simulink model "parrotMinidroneWaypointFollower"  (R2020a)
settings: Solver=ode3  StartTime=0  StopTime=TFinal  FixedStep=Ts  RelTol=1e-3  EnableMultiTasking=on
undefined symbols (not defined in the file): Command, Fault_Category, ft, gcbh, init, m, Rec, s, SDTV, sensorCalibrationData, Sensors, sigbuilder_block, States, stop_time, takeOffDuration, Ts, Vehicle, vrmfunc, VTs
libraries: simulink x16, aerolibconvert2 x4, environmentLibrary x2, visionconversions x2, visiongeotforms x2, aerolibutil x2, aerolibanimutils x1, aerolibnav x1, vrlib x1
(part 4 of 5)

== system parrotMinidroneWaypointFollower/Sensors Model/Sensors (Dynamics)/Sensor System/IMU_Pressure/HAL_acquisition_creator/Gyr Fault Injector1/GyrFI3 ==
  Gyr z : Inport
  Iflag : Inport  Port=2
  Cast To Double : DataTypeConversion  OutDataTypeStr=double
  Cast To Single : DataTypeConversion  OutDataTypeStr=single
  FIBlock : Subsystem  TreatAsAtomicUnit=on  mask(Fault Injector Block){FIBlockName=6, FInjEnable=off, FaultType=Bias/Offset, FaultValue=5, FaultEvent=Deterministic, EventValue=3, FaultEffect=Constant time, EffectValue=2}
      mask prompts: FIBlockName "Number of the FI block instance (e.i. 'name' of the fault injector)"; FInjEnable "Turn on the fault injection for this block"; FaultType "Fault type"; FaultValue "Fault value (bias)"; FaultEvent "Fault injection method"; EventValue "Event value (s)"; FaultEffect "Fault injection effect"; EffectValue "Effect value (s)"
      mask help:
      | This block allows to conduct a fault injection experiment (refer to help if needed).
      | Specify:
      | - name of the block instance.
      | - type of fault: Stuck-at, Package drop, Bias/Offset, Bit flips, Time delay, Noise.
      | - fault event: Failure probability, Mean Time to Failure, Failure Rate Distribution, Deterministic.
      | - fault effect: Once, Constant time, Infinite time, Mean Time to Repair.
      mask init: same as parrotMinidroneWaypointFollower/Sensors Model/Sensors (Dynamics)/Sensor System/IMU_Pressure/HAL_acquisition_creator/Acc Fault Injector/AccFI1/FIBlock
      mask Help:
      | Failure rate distribution is not supported yet!
      | Bit flips, Time delay, and Noise faults may have some bugs :D
      | In different FIBlock instances, the 'name' of the block in GUI must be different (must be an integer number).
      | 
      | Please refer to a comprehensive article regarding the FIBLock: https://flatag.tech/fiblock.html
      | Please cite as: "Fabarisov, T. et al. "Model-based Fault Injection Experiments for the Safety Analysis of Exoskeleton System." Proceedings of the 30th European Safety and Reliability Conference and the 15th Probabilistic Safety Assessment and Management Conference, 2020."
      | 
      | This block allows to conduct a fault injection experiment.
      | Specify:
      | 1) number of the block instance (e.i. 'name' of the fault injector, name shall be unique).
      | 
      | 2) type of fault:
      | - Stuck-at. The block output stays constant, preserving the latest correct value before the error occurrence.
      | - Package drop. The correct output is replaced by the specified Value, emulating a package drop.
      | - Bias/Offset . The defined positive or negative Bias value is added to the block output.
      | - Noise. A random noise value is added. The Boundaries are defined as the percentage of the correct value.
      | - Time delay. A delay is introduced into the signal. During the delay the value is zero.
      | - Bit flips. The defined Number of bits are inverted in the binary representation of the correct value.
      | 
      | 3) fault event:
      | - Failure probability. Errors are injected based on the constant Failure probability for each execution of the block function.
      | - Mean Time to Failure. Errors are injected according to the specified MTTF. Normal distribution.
      | - Deterministic. Уrrors are injected at specific time step.
      | 
      | 4) fault effect:
      | - Once. An error appears only one time during a simulation.
      | - Constant time. The block produces erroneous output during the specified Time period.
      | - Infinite time. The block produces erroneous output until the end of the simulation.
      | - Mean Time to Repair. Normally distributed MTTR regulates the time of the error effect.
      | 
      | FIBlock also provide, what we call, a chained fault injection.
      | Second output of the FIBlock emits a trigger flag.
      | This output signal could be connected to the second input of the FIBlock.
      | In case of the fault injection, this signal will force trigger fault injectionin second FIBlock.
      | 
      | FIBlock supports a base Workspace variables as input in the GUI parameters.
      | 
      | Made By Tagir Fabarisov, TU Dresden 2020
      mask TypeOptions FaultType: Stuck-at | Package drop | Bias/Offset | Bit flips | Time delay | Noise
      mask TypeOptions FaultEvent: Failure probability | Mean Time To Failure | Deterministic
      mask TypeOptions FaultEffect: Once | Constant time | Infinite time | Mean Time To Repair
      mask DialogControl FInjEnable Tooltip: If ticked, then this FIBlock will inject faults
      mask DialogControl Container8 Prompt: Fault type
      mask DialogControl FaultType Tooltip: Specify a type of fault that will be injected
      mask DialogControl FaultTypeDesc Prompt: The defined positive or negative Bias value is added to the block output.
      mask DialogControl Container3 Prompt: Fault injection method
      mask DialogControl Container6 Prompt: Event
      mask DialogControl FaultEvent Tooltip: Specify when fault will be injected
      mask DialogControl FaultEventDesc Prompt: Errors are injected at the specified time
      mask DialogControl Container7 Prompt: Effect
      mask DialogControl FaultEffect Tooltip: Specify how long fault will be injected
      mask DialogControl FaultEffectDesc Prompt: The block produces erroneous output during the specified Time period.
      mask Display:
      | warning off;
      | color('red');
      | a = FaultType;
      | if a == "Sensor: Stuck-at fault"
      |     color('black');
      |     x = linspace(-pi,pi);
      |     y = sin(x);
      |     plot(x,y);
      |     color('red');
      |     disp('        ↯');
      |     x = [-0.7 2];
      |     y = [-0.7 -0.7];
      |     plot(x,y);
      | elseif a == "Network: Package drop"
      |     color('black');
      |     x = linspace(-pi,pi);
      |     y = sin(x);
      |     plot(x,y);
      |     color('red');
      |     disp('        ↯');
      |     x = [-0.7 -0.7];
      |     y = [-0.7 0];
      |     plot(x,y);
      |     x = [-0.7 1];
      |     y = [0 0];
      |     plot(x,y);
      | elseif a == "Sensor: Offset"
      |     color('black');
      |     x1 = linspace(-pi,pi);
      |     y1 = sin(x1)-0.5;
      |     plot(x1,y1);
      |     color('red');
      |     disp('        ↯');
      |     x2 = linspace(0,pi);
      |     y2 = sin(x2);
      |     plot(x2,y2);
      |     x = [0 0];
      |     y = [-0.5 0];
      |     plot(x,y);
      | elseif a == "Hardware: Bit flips"
      |     color('black');
      |     disp('10101010');
      |     color('red');
      |     disp('    0↯');
      | elseif a == "Network: Time delay"
      |     color('black');
      |     x1 = linspace(-pi,pi);
      |     y1 = sin(x1);
      |     plot(x1,y1);
      |     color('red');
      |     disp('        ↯');
      |     x2 = linspace(0,pi);
      |     y2 = sin(x2-0.5);
      |     plot(x2,y2);
      |     x = [0 -0.4];
      |     y = [-0.5 -0.5];
      |     plot(x,y);
      | elseif a == "Sensor: Noise"
      |     color('black');
      |     x1 = linspace(-pi,pi);
      |     y1 = sin(x1);
      |     plot(x1,y1);
      |     color('red');
      |     disp('        ↯');
      |     x = linspace(-pi/8,pi/8,10);
      |     y = sin(x);
      |     for yc = 1:length(y)
      |         d = randi([-2,2])/5;
      |         y(yc) = y(yc) + d;
      |     end
      |     plot(x,y);
      | else
      |     color('red');
      |     disp('Set up Fault Injector!');
      | %Bit flips
      | %Time delay
      | %Noise
      | end
      | warning on;
  z : Outport
  Fflag : Outport  Port=2
  wires:
  Gyr z/1 -> Cast To Double/1
  FIBlock/1(Fdata) -> Cast To Single/1
  Cast To Double/1 -> FIBlock/1(Idata)
  Iflag/1 -> FIBlock/2(Iflag)
  Cast To Single/1 -> z/1
  FIBlock/2(Fflag) -> Fflag/1

== system parrotMinidroneWaypointFollower/Sensors Model/Sensors (Dynamics)/Sensor System/IMU_Pressure/HAL_acquisition_creator/Gyr Fault Injector2/GyrFI1 ==
  Gyr x : Inport
  Iflag : Inport  Port=2
  Cast To Double : DataTypeConversion  OutDataTypeStr=double
  Cast To Single : DataTypeConversion  OutDataTypeStr=single
  FIBlock : Subsystem  TreatAsAtomicUnit=on  mask(Fault Injector Block){FIBlockName=4, FInjEnable=on, FaultType=Bias/Offset, FaultValue=6, FaultEvent=Deterministic, EventValue=4, FaultEffect=Constant time, EffectValue=1.5}
      mask prompts: FIBlockName "Number of the FI block instance (e.i. 'name' of the fault injector)"; FInjEnable "Turn on the fault injection for this block"; FaultType "Fault type"; FaultValue "Fault value (bias)"; FaultEvent "Fault injection method"; EventValue "Event value (s)"; FaultEffect "Fault injection effect"; EffectValue "Effect value (s)"
      mask help:
      | This block allows to conduct a fault injection experiment (refer to help if needed).
      | Specify:
      | - name of the block instance.
      | - type of fault: Stuck-at, Package drop, Bias/Offset, Bit flips, Time delay, Noise.
      | - fault event: Failure probability, Mean Time to Failure, Failure Rate Distribution, Deterministic.
      | - fault effect: Once, Constant time, Infinite time, Mean Time to Repair.
      mask init: same as parrotMinidroneWaypointFollower/Sensors Model/Sensors (Dynamics)/Sensor System/IMU_Pressure/HAL_acquisition_creator/Acc Fault Injector/AccFI1/FIBlock
      mask Help:
      | Failure rate distribution is not supported yet!
      | Bit flips, Time delay, and Noise faults may have some bugs :D
      | In different FIBlock instances, the 'name' of the block in GUI must be different (must be an integer number).
      | 
      | Please refer to a comprehensive article regarding the FIBLock: https://flatag.tech/fiblock.html
      | Please cite as: "Fabarisov, T. et al. "Model-based Fault Injection Experiments for the Safety Analysis of Exoskeleton System." Proceedings of the 30th European Safety and Reliability Conference and the 15th Probabilistic Safety Assessment and Management Conference, 2020."
      | 
      | This block allows to conduct a fault injection experiment.
      | Specify:
      | 1) number of the block instance (e.i. 'name' of the fault injector, name shall be unique).
      | 
      | 2) type of fault:
      | - Stuck-at. The block output stays constant, preserving the latest correct value before the error occurrence.
      | - Package drop. The correct output is replaced by the specified Value, emulating a package drop.
      | - Bias/Offset . The defined positive or negative Bias value is added to the block output.
      | - Noise. A random noise value is added. The Boundaries are defined as the percentage of the correct value.
      | - Time delay. A delay is introduced into the signal. During the delay the value is zero.
      | - Bit flips. The defined Number of bits are inverted in the binary representation of the correct value.
      | 
      | 3) fault event:
      | - Failure probability. Errors are injected based on the constant Failure probability for each execution of the block function.
      | - Mean Time to Failure. Errors are injected according to the specified MTTF. Normal distribution.
      | - Deterministic. Уrrors are injected at specific time step.
      | 
      | 4) fault effect:
      | - Once. An error appears only one time during a simulation.
      | - Constant time. The block produces erroneous output during the specified Time period.
      | - Infinite time. The block produces erroneous output until the end of the simulation.
      | - Mean Time to Repair. Normally distributed MTTR regulates the time of the error effect.
      | 
      | FIBlock also provide, what we call, a chained fault injection.
      | Second output of the FIBlock emits a trigger flag.
      | This output signal could be connected to the second input of the FIBlock.
      | In case of the fault injection, this signal will force trigger fault injectionin second FIBlock.
      | 
      | FIBlock supports a base Workspace variables as input in the GUI parameters.
      | 
      | Made By Tagir Fabarisov, TU Dresden 2020
      mask TypeOptions FaultType: Stuck-at | Package drop | Bias/Offset | Bit flips | Time delay | Noise
      mask TypeOptions FaultEvent: Failure probability | Mean Time To Failure | Deterministic
      mask TypeOptions FaultEffect: Once | Constant time | Infinite time | Mean Time To Repair
      mask DialogControl FInjEnable Tooltip: If ticked, then this FIBlock will inject faults
      mask DialogControl Container8 Prompt: Fault type
      mask DialogControl FaultType Tooltip: Specify a type of fault that will be injected
      mask DialogControl FaultTypeDesc Prompt: The defined positive or negative Bias value is added to the block output.
      mask DialogControl Container3 Prompt: Fault injection method
      mask DialogControl Container6 Prompt: Event
      mask DialogControl FaultEvent Tooltip: Specify when fault will be injected
      mask DialogControl FaultEventDesc Prompt: Errors are injected at the specified time
      mask DialogControl Container7 Prompt: Effect
      mask DialogControl FaultEffect Tooltip: Specify how long fault will be injected
      mask DialogControl FaultEffectDesc Prompt: The block produces erroneous output during the specified Time period.
      mask Display:
      | warning off;
      | color('red');
      | a = FaultType;
      | if a == "Sensor: Stuck-at fault"
      |     color('black');
      |     x = linspace(-pi,pi);
      |     y = sin(x);
      |     plot(x,y);
      |     color('red');
      |     disp('        ↯');
      |     x = [-0.7 2];
      |     y = [-0.7 -0.7];
      |     plot(x,y);
      | elseif a == "Network: Package drop"
      |     color('black');
      |     x = linspace(-pi,pi);
      |     y = sin(x);
      |     plot(x,y);
      |     color('red');
      |     disp('        ↯');
      |     x = [-0.7 -0.7];
      |     y = [-0.7 0];
      |     plot(x,y);
      |     x = [-0.7 1];
      |     y = [0 0];
      |     plot(x,y);
      | elseif a == "Sensor: Offset"
      |     color('black');
      |     x1 = linspace(-pi,pi);
      |     y1 = sin(x1)-0.5;
      |     plot(x1,y1);
      |     color('red');
      |     disp('        ↯');
      |     x2 = linspace(0,pi);
      |     y2 = sin(x2);
      |     plot(x2,y2);
      |     x = [0 0];
      |     y = [-0.5 0];
      |     plot(x,y);
      | elseif a == "Hardware: Bit flips"
      |     color('black');
      |     disp('10101010');
      |     color('red');
      |     disp('    0↯');
      | elseif a == "Network: Time delay"
      |     color('black');
      |     x1 = linspace(-pi,pi);
      |     y1 = sin(x1);
      |     plot(x1,y1);
      |     color('red');
      |     disp('        ↯');
      |     x2 = linspace(0,pi);
      |     y2 = sin(x2-0.5);
      |     plot(x2,y2);
      |     x = [0 -0.4];
      |     y = [-0.5 -0.5];
      |     plot(x,y);
      | elseif a == "Sensor: Noise"
      |     color('black');
      |     x1 = linspace(-pi,pi);
      |     y1 = sin(x1);
      |     plot(x1,y1);
      |     color('red');
      |     disp('        ↯');
      |     x = linspace(-pi/8,pi/8,10);
      |     y = sin(x);
      |     for yc = 1:length(y)
      |         d = randi([-2,2])/5;
      |         y(yc) = y(yc) + d;
      |     end
      |     plot(x,y);
      | else
      |     color('red');
      |     disp('Set up Fault Injector!');
      | %Bit flips
      | %Time delay
      | %Noise
      | end
      | warning on;
  Fflag : Outport
  x : Outport  Port=2
  wires:
  Gyr x/1 -> Cast To Double/1
  FIBlock/1(Fdata) -> Cast To Single/1
  Cast To Double/1 -> FIBlock/1(Idata)
  Iflag/1 -> FIBlock/2(Iflag)
  Cast To Single/1 -> x/1
  FIBlock/2(Fflag) -> Fflag/1

== system parrotMinidroneWaypointFollower/Sensors Model/Sensors (Dynamics)/Sensor System/IMU_Pressure/HAL_acquisition_creator/Gyr Fault Injector2/GyrFI2 ==
  Gyr y : Inport
  Iflag : Inport  Port=2
  Cast To Double : DataTypeConversion  OutDataTypeStr=double
  Cast To Single : DataTypeConversion  OutDataTypeStr=single
  FIBlock : Subsystem  TreatAsAtomicUnit=on  mask(Fault Injector Block){FIBlockName=5, FInjEnable=off, FaultType=Bias/Offset, FaultValue=6, FaultEvent=Deterministic, EventValue=3, FaultEffect=Constant time, EffectValue=2}
      mask prompts: FIBlockName "Number of the FI block instance (e.i. 'name' of the fault injector)"; FInjEnable "Turn on the fault injection for this block"; FaultType "Fault type"; FaultValue "Fault value (bias)"; FaultEvent "Fault injection method"; EventValue "Event value (s)"; FaultEffect "Fault injection effect"; EffectValue "Effect value (s)"
      mask help:
      | This block allows to conduct a fault injection experiment (refer to help if needed).
      | Specify:
      | - name of the block instance.
      | - type of fault: Stuck-at, Package drop, Bias/Offset, Bit flips, Time delay, Noise.
      | - fault event: Failure probability, Mean Time to Failure, Failure Rate Distribution, Deterministic.
      | - fault effect: Once, Constant time, Infinite time, Mean Time to Repair.
      mask init: same as parrotMinidroneWaypointFollower/Sensors Model/Sensors (Dynamics)/Sensor System/IMU_Pressure/HAL_acquisition_creator/Acc Fault Injector/AccFI1/FIBlock
      mask Help:
      | Failure rate distribution is not supported yet!
      | Bit flips, Time delay, and Noise faults may have some bugs :D
      | In different FIBlock instances, the 'name' of the block in GUI must be different (must be an integer number).
      | 
      | Please refer to a comprehensive article regarding the FIBLock: https://flatag.tech/fiblock.html
      | Please cite as: "Fabarisov, T. et al. "Model-based Fault Injection Experiments for the Safety Analysis of Exoskeleton System." Proceedings of the 30th European Safety and Reliability Conference and the 15th Probabilistic Safety Assessment and Management Conference, 2020."
      | 
      | This block allows to conduct a fault injection experiment.
      | Specify:
      | 1) number of the block instance (e.i. 'name' of the fault injector, name shall be unique).
      | 
      | 2) type of fault:
      | - Stuck-at. The block output stays constant, preserving the latest correct value before the error occurrence.
      | - Package drop. The correct output is replaced by the specified Value, emulating a package drop.
      | - Bias/Offset . The defined positive or negative Bias value is added to the block output.
      | - Noise. A random noise value is added. The Boundaries are defined as the percentage of the correct value.
      | - Time delay. A delay is introduced into the signal. During the delay the value is zero.
      | - Bit flips. The defined Number of bits are inverted in the binary representation of the correct value.
      | 
      | 3) fault event:
      | - Failure probability. Errors are injected based on the constant Failure probability for each execution of the block function.
      | - Mean Time to Failure. Errors are injected according to the specified MTTF. Normal distribution.
      | - Deterministic. Уrrors are injected at specific time step.
      | 
      | 4) fault effect:
      | - Once. An error appears only one time during a simulation.
      | - Constant time. The block produces erroneous output during the specified Time period.
      | - Infinite time. The block produces erroneous output until the end of the simulation.
      | - Mean Time to Repair. Normally distributed MTTR regulates the time of the error effect.
      | 
      | FIBlock also provide, what we call, a chained fault injection.
      | Second output of the FIBlock emits a trigger flag.
      | This output signal could be connected to the second input of the FIBlock.
      | In case of the fault injection, this signal will force trigger fault injectionin second FIBlock.
      | 
      | FIBlock supports a base Workspace variables as input in the GUI parameters.
      | 
      | Made By Tagir Fabarisov, TU Dresden 2020
      mask TypeOptions FaultType: Stuck-at | Package drop | Bias/Offset | Bit flips | Time delay | Noise
      mask TypeOptions FaultEvent: Failure probability | Mean Time To Failure | Deterministic
      mask TypeOptions FaultEffect: Once | Constant time | Infinite time | Mean Time To Repair
      mask DialogControl FInjEnable Tooltip: If ticked, then this FIBlock will inject faults
      mask DialogControl Container8 Prompt: Fault type
      mask DialogControl FaultType Tooltip: Specify a type of fault that will be injected
      mask DialogControl FaultTypeDesc Prompt: The defined positive or negative Bias value is added to the block output.
      mask DialogControl Container3 Prompt: Fault injection method
      mask DialogControl Container6 Prompt: Event
      mask DialogControl FaultEvent Tooltip: Specify when fault will be injected
      mask DialogControl FaultEventDesc Prompt: Errors are injected at the specified time
      mask DialogControl Container7 Prompt: Effect
      mask DialogControl FaultEffect Tooltip: Specify how long fault will be injected
      mask DialogControl FaultEffectDesc Prompt: The block produces erroneous output during the specified Time period.
      mask Display:
      | warning off;
      | color('red');
      | a = FaultType;
      | if a == "Sensor: Stuck-at fault"
      |     color('black');
      |     x = linspace(-pi,pi);
      |     y = sin(x);
      |     plot(x,y);
      |     color('red');
      |     disp('        ↯');
      |     x = [-0.7 2];
      |     y = [-0.7 -0.7];
      |     plot(x,y);
      | elseif a == "Network: Package drop"
      |     color('black');
      |     x = linspace(-pi,pi);
      |     y = sin(x);
      |     plot(x,y);
      |     color('red');
      |     disp('        ↯');
      |     x = [-0.7 -0.7];
      |     y = [-0.7 0];
      |     plot(x,y);
      |     x = [-0.7 1];
      |     y = [0 0];
      |     plot(x,y);
      | elseif a == "Sensor: Offset"
      |     color('black');
      |     x1 = linspace(-pi,pi);
      |     y1 = sin(x1)-0.5;
      |     plot(x1,y1);
      |     color('red');
      |     disp('        ↯');
      |     x2 = linspace(0,pi);
      |     y2 = sin(x2);
      |     plot(x2,y2);
      |     x = [0 0];
      |     y = [-0.5 0];
      |     plot(x,y);
      | elseif a == "Hardware: Bit flips"
      |     color('black');
      |     disp('10101010');
      |     color('red');
      |     disp('    0↯');
      | elseif a == "Network: Time delay"
      |     color('black');
      |     x1 = linspace(-pi,pi);
      |     y1 = sin(x1);
      |     plot(x1,y1);
      |     color('red');
      |     disp('        ↯');
      |     x2 = linspace(0,pi);
      |     y2 = sin(x2-0.5);
      |     plot(x2,y2);
      |     x = [0 -0.4];
      |     y = [-0.5 -0.5];
      |     plot(x,y);
      | elseif a == "Sensor: Noise"
      |     color('black');
      |     x1 = linspace(-pi,pi);
      |     y1 = sin(x1);
      |     plot(x1,y1);
      |     color('red');
      |     disp('        ↯');
      |     x = linspace(-pi/8,pi/8,10);
      |     y = sin(x);
      |     for yc = 1:length(y)
      |         d = randi([-2,2])/5;
      |         y(yc) = y(yc) + d;
      |     end
      |     plot(x,y);
      | else
      |     color('red');
      |     disp('Set up Fault Injector!');
      | %Bit flips
      | %Time delay
      | %Noise
      | end
      | warning on;
  Fflag : Outport
  y : Outport  Port=2
  wires:
  Gyr y/1 -> Cast To Double/1
  FIBlock/1(Fdata) -> Cast To Single/1
  Cast To Double/1 -> FIBlock/1(Idata)
  Iflag/1 -> FIBlock/2(Iflag)
  Cast To Single/1 -> y/1
  FIBlock/2(Fflag) -> Fflag/1

== system parrotMinidroneWaypointFollower/Sensors Model/Sensors (Dynamics)/Sensor System/IMU_Pressure/HAL_acquisition_creator/Gyr Fault Injector2/GyrFI3 ==
  Gyr z : Inport
  Iflag : Inport  Port=2
  Cast To Double : DataTypeConversion  OutDataTypeStr=double
  Cast To Single : DataTypeConversion  OutDataTypeStr=single
  FIBlock : Subsystem  TreatAsAtomicUnit=on  mask(Fault Injector Block){FIBlockName=6, FInjEnable=off, FaultType=Bias/Offset, FaultValue=5, FaultEvent=Deterministic, EventValue=3, FaultEffect=Constant time, EffectValue=2}
      mask prompts: FIBlockName "Number of the FI block instance (e.i. 'name' of the fault injector)"; FInjEnable "Turn on the fault injection for this block"; FaultType "Fault type"; FaultValue "Fault value (bias)"; FaultEvent "Fault injection method"; EventValue "Event value (s)"; FaultEffect "Fault injection effect"; EffectValue "Effect value (s)"
      mask help:
      | This block allows to conduct a fault injection experiment (refer to help if needed).
      | Specify:
      | - name of the block instance.
      | - type of fault: Stuck-at, Package drop, Bias/Offset, Bit flips, Time delay, Noise.
      | - fault event: Failure probability, Mean Time to Failure, Failure Rate Distribution, Deterministic.
      | - fault effect: Once, Constant time, Infinite time, Mean Time to Repair.
      mask init: same as parrotMinidroneWaypointFollower/Sensors Model/Sensors (Dynamics)/Sensor System/IMU_Pressure/HAL_acquisition_creator/Acc Fault Injector/AccFI1/FIBlock
      mask Help:
      | Failure rate distribution is not supported yet!
      | Bit flips, Time delay, and Noise faults may have some bugs :D
      | In different FIBlock instances, the 'name' of the block in GUI must be different (must be an integer number).
      | 
      | Please refer to a comprehensive article regarding the FIBLock: https://flatag.tech/fiblock.html
      | Please cite as: "Fabarisov, T. et al. "Model-based Fault Injection Experiments for the Safety Analysis of Exoskeleton System." Proceedings of the 30th European Safety and Reliability Conference and the 15th Probabilistic Safety Assessment and Management Conference, 2020."
      | 
      | This block allows to conduct a fault injection experiment.
      | Specify:
      | 1) number of the block instance (e.i. 'name' of the fault injector, name shall be unique).
      | 
      | 2) type of fault:
      | - Stuck-at. The block output stays constant, preserving the latest correct value before the error occurrence.
      | - Package drop. The correct output is replaced by the specified Value, emulating a package drop.
      | - Bias/Offset . The defined positive or negative Bias value is added to the block output.
      | - Noise. A random noise value is added. The Boundaries are defined as the percentage of the correct value.
      | - Time delay. A delay is introduced into the signal. During the delay the value is zero.
      | - Bit flips. The defined Number of bits are inverted in the binary representation of the correct value.
      | 
      | 3) fault event:
      | - Failure probability. Errors are injected based on the constant Failure probability for each execution of the block function.
      | - Mean Time to Failure. Errors are injected according to the specified MTTF. Normal distribution.
      | - Deterministic. Уrrors are injected at specific time step.
      | 
      | 4) fault effect:
      | - Once. An error appears only one time during a simulation.
      | - Constant time. The block produces erroneous output during the specified Time period.
      | - Infinite time. The block produces erroneous output until the end of the simulation.
      | - Mean Time to Repair. Normally distributed MTTR regulates the time of the error effect.
      | 
      | FIBlock also provide, what we call, a chained fault injection.
      | Second output of the FIBlock emits a trigger flag.
      | This output signal could be connected to the second input of the FIBlock.
      | In case of the fault injection, this signal will force trigger fault injectionin second FIBlock.
      | 
      | FIBlock supports a base Workspace variables as input in the GUI parameters.
      | 
      | Made By Tagir Fabarisov, TU Dresden 2020
      mask TypeOptions FaultType: Stuck-at | Package drop | Bias/Offset | Bit flips | Time delay | Noise
      mask TypeOptions FaultEvent: Failure probability | Mean Time To Failure | Deterministic
      mask TypeOptions FaultEffect: Once | Constant time | Infinite time | Mean Time To Repair
      mask DialogControl FInjEnable Tooltip: If ticked, then this FIBlock will inject faults
      mask DialogControl Container8 Prompt: Fault type
      mask DialogControl FaultType Tooltip: Specify a type of fault that will be injected
      mask DialogControl FaultTypeDesc Prompt: The defined positive or negative Bias value is added to the block output.
      mask DialogControl Container3 Prompt: Fault injection method
      mask DialogControl Container6 Prompt: Event
      mask DialogControl FaultEvent Tooltip: Specify when fault will be injected
      mask DialogControl FaultEventDesc Prompt: Errors are injected at the specified time
      mask DialogControl Container7 Prompt: Effect
      mask DialogControl FaultEffect Tooltip: Specify how long fault will be injected
      mask DialogControl FaultEffectDesc Prompt: The block produces erroneous output during the specified Time period.
      mask Display:
      | warning off;
      | color('red');
      | a = FaultType;
      | if a == "Sensor: Stuck-at fault"
      |     color('black');
      |     x = linspace(-pi,pi);
      |     y = sin(x);
      |     plot(x,y);
      |     color('red');
      |     disp('        ↯');
      |     x = [-0.7 2];
      |     y = [-0.7 -0.7];
      |     plot(x,y);
      | elseif a == "Network: Package drop"
      |     color('black');
      |     x = linspace(-pi,pi);
      |     y = sin(x);
      |     plot(x,y);
      |     color('red');
      |     disp('        ↯');
      |     x = [-0.7 -0.7];
      |     y = [-0.7 0];
      |     plot(x,y);
      |     x = [-0.7 1];
      |     y = [0 0];
      |     plot(x,y);
      | elseif a == "Sensor: Offset"
      |     color('black');
      |     x1 = linspace(-pi,pi);
      |     y1 = sin(x1)-0.5;
      |     plot(x1,y1);
      |     color('red');
      |     disp('        ↯');
      |     x2 = linspace(0,pi);
      |     y2 = sin(x2);
      |     plot(x2,y2);
      |     x = [0 0];
      |     y = [-0.5 0];
      |     plot(x,y);
      | elseif a == "Hardware: Bit flips"
      |     color('black');
      |     disp('10101010');
      |     color('red');
      |     disp('    0↯');
      | elseif a == "Network: Time delay"
      |     color('black');
      |     x1 = linspace(-pi,pi);
      |     y1 = sin(x1);
      |     plot(x1,y1);
      |     color('red');
      |     disp('        ↯');
      |     x2 = linspace(0,pi);
      |     y2 = sin(x2-0.5);
      |     plot(x2,y2);
      |     x = [0 -0.4];
      |     y = [-0.5 -0.5];
      |     plot(x,y);
      | elseif a == "Sensor: Noise"
      |     color('black');
      |     x1 = linspace(-pi,pi);
      |     y1 = sin(x1);
      |     plot(x1,y1);
      |     color('red');
      |     disp('        ↯');
      |     x = linspace(-pi/8,pi/8,10);
      |     y = sin(x);
      |     for yc = 1:length(y)
      |         d = randi([-2,2])/5;
      |         y(yc) = y(yc) + d;
      |     end
      |     plot(x,y);
      | else
      |     color('red');
      |     disp('Set up Fault Injector!');
      | %Bit flips
      | %Time delay
      | %Noise
      | end
      | warning on;
  z : Outport
  Fflag : Outport  Port=2
  wires:
  Gyr z/1 -> Cast To Double/1
  FIBlock/1(Fdata) -> Cast To Single/1
  Cast To Double/1 -> FIBlock/1(Idata)
  Iflag/1 -> FIBlock/2(Iflag)
  Cast To Single/1 -> z/1
  FIBlock/2(Fflag) -> Fflag/1

== system parrotMinidroneWaypointFollower/Sensors Model/Sensors (Dynamics)/Sensor System/IMU_Pressure/HAL_acquisition_creator/HAL_ultrasound_SI_creator/HAL_list_echo_t_creator ==
  Bus Creator7 : BusCreator  Inputs=2  OutDataTypeStr=Bus: HAL_list_echo_t  NonVirtualBus=on
  HAL_echo_t_creator : Subsystem
  Vector Concatenate : Concatenate  NumInputs=30
  number_of_echoes : Constant  Value=0  OutDataTypeStr=uint8
  HAL_list_echo : Outport  VectorParamsAs1DForOutWhenUnconnected=off
  wires:
  HAL_echo_t_creator/1(HAL_echo_t) -> Vector Concatenate/1, Vector Concatenate/2, Vector Concatenate/3, Vector Concatenate/4, Vector Concatenate/5, Vector Concatenate/6, Vector Concatenate/7, Vector Concatenate/8, Vector Concatenate/9, Vector Concatenate/10, Vector Concatenate/11, Vector Concatenate/12, Vector Concatenate/13, Vector Concatenate/14, Vector Concatenate/15, Vector Concatenate/16, Vector Concatenate/17, Vector Concatenate/18, Vector Concatenate/19, Vector Concatenate/20, Vector Concatenate/21, Vector Concatenate/22, Vector Concatenate/23, Vector Concatenate/24, Vector Concatenate/25, Vector Concatenate/26, Vector Concatenate/27, Vector Concatenate/28, Vector Concatenate/29, Vector Concatenate/30
  Vector Concatenate/1 -> Bus Creator7/1  "tab_echo"
  Bus Creator7/1 -> HAL_list_echo/1  "HAL_list_echo"
  number_of_echoes/1 -> Bus Creator7/2  "number_of_echoes"

== system parrotMinidroneWaypointFollower/Sensors Model/Sensors (Dynamics)/Sensor System/IMU_Pressure/HAL_acquisition_creator/HAL_ultrasound_SI_creator/HAL_list_echo_t_creator1 ==
  Bus Creator7 : BusCreator  Inputs=2  OutDataTypeStr=Bus: HAL_list_echo_t  NonVirtualBus=on
  HAL_echo_t_creator : Subsystem
  Vector Concatenate : Concatenate  NumInputs=30
  number_of_echoes : Constant  Value=0  OutDataTypeStr=uint8
  HAL_list_echo : Outport  VectorParamsAs1DForOutWhenUnconnected=off
  wires:
  number_of_echoes/1 -> Bus Creator7/2  "number_of_echoes"
  Bus Creator7/1 -> HAL_list_echo/1  "HAL_list_echo"
  Vector Concatenate/1 -> Bus Creator7/1  "tab_echo"
  HAL_echo_t_creator/1(HAL_echo_t) -> Vector Concatenate/30, Vector Concatenate/29, Vector Concatenate/28, Vector Concatenate/27, Vector Concatenate/26, Vector Concatenate/25, Vector Concatenate/24, Vector Concatenate/23, Vector Concatenate/22, Vector Concatenate/21, Vector Concatenate/20, Vector Concatenate/19, Vector Concatenate/18, Vector Concatenate/17, Vector Concatenate/16, Vector Concatenate/15, Vector Concatenate/14, Vector Concatenate/13, Vector Concatenate/12, Vector Concatenate/11, Vector Concatenate/10, Vector Concatenate/9, Vector Concatenate/8, Vector Concatenate/7, Vector Concatenate/6, Vector Concatenate/5, Vector Concatenate/4, Vector Concatenate/3, Vector Concatenate/2, Vector Concatenate/1

== system parrotMinidroneWaypointFollower/Sensors Model/Sensors (Feedthrough)/Sensor System/IMU_Pressure/HAL_acquisition_creator/HAL_ultrasound_SI_creator/HAL_list_echo_t_creator ==
  Bus Creator7 : BusCreator  Inputs=2  OutDataTypeStr=Bus: HAL_list_echo_t  NonVirtualBus=on
  HAL_echo_t_creator : Subsystem
  Vector Concatenate : Concatenate  NumInputs=30
  number_of_echoes : Constant  Value=0  OutDataTypeStr=uint8
  HAL_list_echo : Outport  VectorParamsAs1DForOutWhenUnconnected=off
  wires:
  HAL_echo_t_creator/1(HAL_echo_t) -> Vector Concatenate/1, Vector Concatenate/2, Vector Concatenate/3, Vector Concatenate/4, Vector Concatenate/5, Vector Concatenate/6, Vector Concatenate/7, Vector Concatenate/8, Vector Concatenate/9, Vector Concatenate/10, Vector Concatenate/11, Vector Concatenate/12, Vector Concatenate/13, Vector Concatenate/14, Vector Concatenate/15, Vector Concatenate/16, Vector Concatenate/17, Vector Concatenate/18, Vector Concatenate/19, Vector Concatenate/20, Vector Concatenate/21, Vector Concatenate/22, Vector Concatenate/23, Vector Concatenate/24, Vector Concatenate/25, Vector Concatenate/26, Vector Concatenate/27, Vector Concatenate/28, Vector Concatenate/29, Vector Concatenate/30
  Vector Concatenate/1 -> Bus Creator7/1  "tab_echo"
  Bus Creator7/1 -> HAL_list_echo/1  "HAL_list_echo"
  number_of_echoes/1 -> Bus Creator7/2  "number_of_echoes"

== system parrotMinidroneWaypointFollower/Sensors Model/Sensors (Feedthrough)/Sensor System/IMU_Pressure/HAL_acquisition_creator/HAL_ultrasound_SI_creator/HAL_list_echo_t_creator1 ==
  Bus Creator7 : BusCreator  Inputs=2  OutDataTypeStr=Bus: HAL_list_echo_t  NonVirtualBus=on
  HAL_echo_t_creator : Subsystem
  Vector Concatenate : Concatenate  NumInputs=30
  number_of_echoes : Constant  Value=0  OutDataTypeStr=uint8
  HAL_list_echo : Outport  VectorParamsAs1DForOutWhenUnconnected=off
  wires:
  number_of_echoes/1 -> Bus Creator7/2  "number_of_echoes"
  Bus Creator7/1 -> HAL_list_echo/1  "HAL_list_echo"
  Vector Concatenate/1 -> Bus Creator7/1  "tab_echo"
  HAL_echo_t_creator/1(HAL_echo_t) -> Vector Concatenate/30, Vector Concatenate/29, Vector Concatenate/28, Vector Concatenate/27, Vector Concatenate/26, Vector Concatenate/25, Vector Concatenate/24, Vector Concatenate/23, Vector Concatenate/22, Vector Concatenate/21, Vector Concatenate/20, Vector Concatenate/19, Vector Concatenate/18, Vector Concatenate/17, Vector Concatenate/16, Vector Concatenate/15, Vector Concatenate/14, Vector Concatenate/13, Vector Concatenate/12, Vector Concatenate/11, Vector Concatenate/10, Vector Concatenate/9, Vector Concatenate/8, Vector Concatenate/7, Vector Concatenate/6, Vector Concatenate/5, Vector Concatenate/4, Vector Concatenate/3, Vector Concatenate/2, Vector Concatenate/1

== system parrotMinidroneWaypointFollower/Sensors Model/Sensors (Dynamics)/Sensor System/IMU_Pressure/HAL_acquisition_creator/Acc Fault Injector/AccFI1/FIBlock ==
  Idata : Inport
  Iflag : Inport  Port=2
  Clock : Clock
  Constant0 : Constant  Value=0
  Constant1 : Constant
  FaultInjectionBlock : MATLAB Function  TreatAsAtomicUnit=on
  Switch : Switch  Criteria=u2 > Threshold
  Fdata : Outport
  Fflag : Outport  Port=2
  wires:
  Switch/1 -> Fflag/1
  FaultInjectionBlock/2(error_flag) -> Switch/2
  Constant1/1 -> Switch/1
  Constant0/1 -> Switch/3
  Iflag/1 -> FaultInjectionBlock/3(input_flag)
  FaultInjectionBlock/1(error_data) -> Fdata/1
  Clock/1 -> FaultInjectionBlock/1(time)
  Idata/1 -> FaultInjectionBlock/2(data)

== system parrotMinidroneWaypointFollower/Sensors Model/Sensors (Dynamics)/Sensor System/IMU_Pressure/HAL_acquisition_creator/Acc Fault Injector/AccFI2/FIBlock ==
  Idata : Inport
  Iflag : Inport  Port=2
  Clock : Clock
  Constant0 : Constant  Value=0
  Constant1 : Constant
  FaultInjectionBlock : MATLAB Function  TreatAsAtomicUnit=on
  Switch : Switch  Criteria=u2 > Threshold
  Fdata : Outport
  Fflag : Outport  Port=2
  wires:
  Switch/1 -> Fflag/1
  FaultInjectionBlock/2(error_flag) -> Switch/2
  Constant1/1 -> Switch/1
  Constant0/1 -> Switch/3
  Iflag/1 -> FaultInjectionBlock/3(input_flag)
  FaultInjectionBlock/1(error_data) -> Fdata/1
  Clock/1 -> FaultInjectionBlock/1(time)
  Idata/1 -> FaultInjectionBlock/2(data)

== system parrotMinidroneWaypointFollower/Sensors Model/Sensors (Dynamics)/Sensor System/IMU_Pressure/HAL_acquisition_creator/Acc Fault Injector/AccFI3/FIBlock ==
  Idata : Inport
  Iflag : Inport  Port=2
  Clock : Clock
  Constant0 : Constant  Value=0
  Constant1 : Constant
  FaultInjectionBlock : MATLAB Function  TreatAsAtomicUnit=on
  Switch : Switch  Criteria=u2 > Threshold
  Fdata : Outport
  Fflag : Outport  Port=2
  wires:
  Switch/1 -> Fflag/1
  FaultInjectionBlock/2(error_flag) -> Switch/2
  Constant1/1 -> Switch/1
  Constant0/1 -> Switch/3
  Iflag/1 -> FaultInjectionBlock/3(input_flag)
  FaultInjectionBlock/1(error_data) -> Fdata/1
  Clock/1 -> FaultInjectionBlock/1(time)
  Idata/1 -> FaultInjectionBlock/2(data)

== system parrotMinidroneWaypointFollower/Sensors Model/Sensors (Dynamics)/Sensor System/IMU_Pressure/HAL_acquisition_creator/Gyr Fault Injector1/GyrFI1/FIBlock ==
  Idata : Inport
  Iflag : Inport  Port=2
  Clock : Clock
  Constant0 : Constant  Value=0
  Constant1 : Constant
  FaultInjectionBlock : MATLAB Function  TreatAsAtomicUnit=on
  Switch : Switch  Criteria=u2 > Threshold
  Fdata : Outport
  Fflag : Outport  Port=2
  wires:
  Switch/1 -> Fflag/1
  FaultInjectionBlock/2(error_flag) -> Switch/2
  Constant1/1 -> Switch/1
  Constant0/1 -> Switch/3
  Iflag/1 -> FaultInjectionBlock/3(input_flag)
  FaultInjectionBlock/1(error_data) -> Fdata/1
  Clock/1 -> FaultInjectionBlock/1(time)
  Idata/1 -> FaultInjectionBlock/2(data)

== system parrotMinidroneWaypointFollower/Sensors Model/Sensors (Dynamics)/Sensor System/IMU_Pressure/HAL_acquisition_creator/Gyr Fault Injector1/GyrFI2/FIBlock ==
  Idata : Inport
  Iflag : Inport  Port=2
  Clock : Clock
  Constant0 : Constant  Value=0
  Constant1 : Constant
  FaultInjectionBlock : MATLAB Function  TreatAsAtomicUnit=on
  Switch : Switch  Criteria=u2 > Threshold
  Fdata : Outport
  Fflag : Outport  Port=2
  wires:
  Switch/1 -> Fflag/1
  FaultInjectionBlock/2(error_flag) -> Switch/2
  Constant1/1 -> Switch/1
  Constant0/1 -> Switch/3
  Iflag/1 -> FaultInjectionBlock/3(input_flag)
  FaultInjectionBlock/1(error_data) -> Fdata/1
  Clock/1 -> FaultInjectionBlock/1(time)
  Idata/1 -> FaultInjectionBlock/2(data)

== system parrotMinidroneWaypointFollower/Sensors Model/Sensors (Dynamics)/Sensor System/IMU_Pressure/HAL_acquisition_creator/Gyr Fault Injector1/GyrFI3/FIBlock ==
  Idata : Inport
  Iflag : Inport  Port=2
  Clock : Clock
  Constant0 : Constant  Value=0
  Constant1 : Constant
  FaultInjectionBlock : MATLAB Function  TreatAsAtomicUnit=on
  Switch : Switch  Criteria=u2 > Threshold
  Fdata : Outport
  Fflag : Outport  Port=2
  wires:
  Switch/1 -> Fflag/1
  FaultInjectionBlock/2(error_flag) -> Switch/2
  Constant1/1 -> Switch/1
  Constant0/1 -> Switch/3
  Iflag/1 -> FaultInjectionBlock/3(input_flag)
  FaultInjectionBlock/1(error_data) -> Fdata/1
  Clock/1 -> FaultInjectionBlock/1(time)
  Idata/1 -> FaultInjectionBlock/2(data)

== system parrotMinidroneWaypointFollower/Sensors Model/Sensors (Dynamics)/Sensor System/IMU_Pressure/HAL_acquisition_creator/Gyr Fault Injector2/GyrFI1/FIBlock ==
  Idata : Inport
  Iflag : Inport  Port=2
  Clock : Clock
  Constant0 : Constant  Value=0
  Constant1 : Constant
  FaultInjectionBlock : MATLAB Function  TreatAsAtomicUnit=on
  Switch : Switch  Criteria=u2 > Threshold
  Fdata : Outport
  Fflag : Outport  Port=2
  wires:
  Switch/1 -> Fflag/1
  FaultInjectionBlock/2(error_flag) -> Switch/2
  Constant1/1 -> Switch/1
  Constant0/1 -> Switch/3
  Iflag/1 -> FaultInjectionBlock/3(input_flag)
  FaultInjectionBlock/1(error_data) -> Fdata/1
  Clock/1 -> FaultInjectionBlock/1(time)
  Idata/1 -> FaultInjectionBlock/2(data)

== system parrotMinidroneWaypointFollower/Sensors Model/Sensors (Dynamics)/Sensor System/IMU_Pressure/HAL_acquisition_creator/Gyr Fault Injector2/GyrFI2/FIBlock ==
  Idata : Inport
  Iflag : Inport  Port=2
  Clock : Clock
  Constant0 : Constant  Value=0
  Constant1 : Constant
  FaultInjectionBlock : MATLAB Function  TreatAsAtomicUnit=on
  Switch : Switch  Criteria=u2 > Threshold
  Fdata : Outport
  Fflag : Outport  Port=2
  wires:
  Switch/1 -> Fflag/1
  FaultInjectionBlock/2(error_flag) -> Switch/2
  Constant1/1 -> Switch/1
  Constant0/1 -> Switch/3
  Iflag/1 -> FaultInjectionBlock/3(input_flag)
  FaultInjectionBlock/1(error_data) -> Fdata/1
  Clock/1 -> FaultInjectionBlock/1(time)
  Idata/1 -> FaultInjectionBlock/2(data)

== system parrotMinidroneWaypointFollower/Sensors Model/Sensors (Dynamics)/Sensor System/IMU_Pressure/HAL_acquisition_creator/Gyr Fault Injector2/GyrFI3/FIBlock ==
  Idata : Inport
  Iflag : Inport  Port=2
  Clock : Clock
  Constant0 : Constant  Value=0
  Constant1 : Constant
  FaultInjectionBlock : MATLAB Function  TreatAsAtomicUnit=on
  Switch : Switch  Criteria=u2 > Threshold
  Fdata : Outport
  Fflag : Outport  Port=2
  wires:
  Switch/1 -> Fflag/1
  FaultInjectionBlock/2(error_flag) -> Switch/2
  Constant1/1 -> Switch/1
  Constant0/1 -> Switch/3
  Iflag/1 -> FaultInjectionBlock/3(input_flag)
  FaultInjectionBlock/1(error_data) -> Fdata/1
  Clock/1 -> FaultInjectionBlock/1(time)
  Idata/1 -> FaultInjectionBlock/2(data)

== system parrotMinidroneWaypointFollower/Sensors Model/Sensors (Dynamics)/Sensor System/IMU_Pressure/HAL_acquisition_creator/HAL_ultrasound_SI_creator/HAL_list_echo_t_creator/HAL_echo_t_creator ==
  Bus Creator6 : BusCreator  Inputs=7  OutDataTypeStr=Bus: HAL_echo_t  NonVirtualBus=on
  begin_echo_index{,1,4,6} (4 alike) : Constant  Value=0  OutDataTypeStr=uint16
  begin_echo_index2 : Constant  Value=0  OutDataTypeStr=int16
  begin_echo_index3 : Constant  Value=0  OutDataTypeStr=int32
  begin_echo_index5 : Constant  Value=0  OutDataTypeStr=int16
  HAL_echo_t : Outport  OutDataTypeStr=Bus: HAL_echo_t  VectorParamsAs1DForOutWhenUnconnected=off
  wires:
  begin_echo_index6/1 -> Bus Creator6/7  "pre_max_index"
  begin_echo_index5/1 -> Bus Creator6/6  "d_echo"
  begin_echo_index4/1 -> Bus Creator6/5  "precedent"
  begin_echo_index3/1 -> Bus Creator6/4  "max_value"
  begin_echo_index2/1 -> Bus Creator6/3  "max_value_index"
  begin_echo_index1/1 -> Bus Creator6/2  "end_echo_index"
  begin_echo_index/1 -> Bus Creator6/1  "begin_echo_index"
  Bus Creator6/1 -> HAL_echo_t/1  "HAL_echo_t"

== system parrotMinidroneWaypointFollower/Sensors Model/Sensors (Dynamics)/Sensor System/IMU_Pressure/HAL_acquisition_creator/HAL_ultrasound_SI_creator/HAL_list_echo_t_creator1/HAL_echo_t_creator ==
  Bus Creator6 : BusCreator  Inputs=7  OutDataTypeStr=Bus: HAL_echo_t  NonVirtualBus=on
  begin_echo_index{,1,4,6} (4 alike) : Constant  Value=0  OutDataTypeStr=uint16
  begin_echo_index2 : Constant  Value=0  OutDataTypeStr=int16
  begin_echo_index3 : Constant  Value=0  OutDataTypeStr=int32
  begin_echo_index5 : Constant  Value=0  OutDataTypeStr=int16
  HAL_echo_t : Outport  OutDataTypeStr=Bus: HAL_echo_t  VectorParamsAs1DForOutWhenUnconnected=off
  wires:
  Bus Creator6/1 -> HAL_echo_t/1  "HAL_echo_t"
  begin_echo_index/1 -> Bus Creator6/1  "begin_echo_index"
  begin_echo_index1/1 -> Bus Creator6/2  "end_echo_index"
  begin_echo_index2/1 -> Bus Creator6/3  "max_value_index"
  begin_echo_index3/1 -> Bus Creator6/4  "max_value"
  begin_echo_index4/1 -> Bus Creator6/5  "precedent"
  begin_echo_index5/1 -> Bus Creator6/6  "d_echo"
  begin_echo_index6/1 -> Bus Creator6/7  "pre_max_index"

== system parrotMinidroneWaypointFollower/Sensors Model/Sensors (Feedthrough)/Sensor System/IMU_Pressure/HAL_acquisition_creator/HAL_ultrasound_SI_creator/HAL_list_echo_t_creator/HAL_echo_t_creator ==
  Bus Creator6 : BusCreator  Inputs=7  OutDataTypeStr=Bus: HAL_echo_t  NonVirtualBus=on
  begin_echo_index{,1,4,6} (4 alike) : Constant  Value=0  OutDataTypeStr=uint16
  begin_echo_index2 : Constant  Value=0  OutDataTypeStr=int16
  begin_echo_index3 : Constant  Value=0  OutDataTypeStr=int32
  begin_echo_index5 : Constant  Value=0  OutDataTypeStr=int16
  HAL_echo_t : Outport  OutDataTypeStr=Bus: HAL_echo_t  VectorParamsAs1DForOutWhenUnconnected=off
  wires:
  begin_echo_index6/1 -> Bus Creator6/7  "pre_max_index"
  begin_echo_index5/1 -> Bus Creator6/6  "d_echo"
  begin_echo_index4/1 -> Bus Creator6/5  "precedent"
  begin_echo_index3/1 -> Bus Creator6/4  "max_value"
  begin_echo_index2/1 -> Bus Creator6/3  "max_value_index"
  begin_echo_index1/1 -> Bus Creator6/2  "end_echo_index"
  begin_echo_index/1 -> Bus Creator6/1  "begin_echo_index"
  Bus Creator6/1 -> HAL_echo_t/1  "HAL_echo_t"

== system parrotMinidroneWaypointFollower/Sensors Model/Sensors (Feedthrough)/Sensor System/IMU_Pressure/HAL_acquisition_creator/HAL_ultrasound_SI_creator/HAL_list_echo_t_creator1/HAL_echo_t_creator ==
  Bus Creator6 : BusCreator  Inputs=7  OutDataTypeStr=Bus: HAL_echo_t  NonVirtualBus=on
  begin_echo_index{,1,4,6} (4 alike) : Constant  Value=0  OutDataTypeStr=uint16
  begin_echo_index2 : Constant  Value=0  OutDataTypeStr=int16
  begin_echo_index3 : Constant  Value=0  OutDataTypeStr=int32
  begin_echo_index5 : Constant  Value=0  OutDataTypeStr=int16
  HAL_echo_t : Outport  OutDataTypeStr=Bus: HAL_echo_t  VectorParamsAs1DForOutWhenUnconnected=off
  wires:
  Bus Creator6/1 -> HAL_echo_t/1  "HAL_echo_t"
  begin_echo_index/1 -> Bus Creator6/1  "begin_echo_index"
  begin_echo_index1/1 -> Bus Creator6/2  "end_echo_index"
  begin_echo_index2/1 -> Bus Creator6/3  "max_value_index"
  begin_echo_index3/1 -> Bus Creator6/4  "max_value"
  begin_echo_index4/1 -> Bus Creator6/5  "precedent"
  begin_echo_index5/1 -> Bus Creator6/6  "d_echo"
  begin_echo_index6/1 -> Bus Creator6/7  "pre_max_index"

== matlab function parrotMinidroneWaypointFollower/Sensors Model/Sensors (Dynamics)/Sensor System/IMU_Pressure/HAL_acquisition_creator/Gyr Fault Injector2/GyrFI3/FIBlock/FaultInjectionBlock ==
  data: time input; error_data output; data input; input_flag input; FIBlockName parameter; error_flag output
function [error_data, error_flag] = fcn(time, data, input_flag, FIBlockName)
coder.extrinsic('wrapper');
d = data;
t = time;
n = num2str(FIBlockName);
f = input_flag;
error_data = coder.nullcopy(zeros(size(d)));
error_flag = 0;
[error_data, error_flag] = wrapper(d, t, n, f);
end

== matlab function parrotMinidroneWaypointFollower/Sensors Model/Sensors (Dynamics)/Sensor System/IMU_Pressure/HAL_acquisition_creator/Acc Fault Injector/AccFI1/FIBlock/FaultInjectionBlock ==
  data: time input; error_data output; data input; input_flag input; FIBlockName parameter; error_flag output
function [error_data, error_flag] = fcn(time, data, input_flag, FIBlockName)
coder.extrinsic('wrapper');
d = data;
t = time;
n = num2str(FIBlockName);
f = input_flag;
error_data = coder.nullcopy(zeros(size(d)));
error_flag = 0;
[error_data, error_flag] = wrapper(d, t, n, f);
end
